simulink model "heat_exchanger_OL"  (R2017b)
settings: Solver=VariableStepAuto  StartTime=0.0  StopTime=200  RelTol=1e-3
values from neighbouring files (symbols this model uses):
  Area = n*A_heat_plate    (= 9.8716)    [heat_exchanger_config.m]    (also in linearization.m = 20)
  cp_H2O = 4190    [heat_exchanger_config.m]    (also in linearization.m)
  cp_wort = 4062    [heat_exchanger_config.m]    (also in linearization.m = 4000)
  HE_delay = 25    [heat_exchanger_config.m]    (also in linearization.m = 5)
  m_H2O = m_wort    (= 10)    [heat_exchanger_config.m]    (also in linearization.m = 1)
  m_wort = 10    [heat_exchanger_config.m]    (also in linearization.m = 1)
  T_H2O_in = 5    [heat_exchanger_config.m]    (also in linearization.m = 10)
  T_wort_in = 95    [heat_exchanger_config.m]    (also in linearization.m = 70)
  U = (m_dot_h_data*cp_wort*(T_wort_in-T_wort_out)*log(Delta_T2/Delta_T1))/     (Area*(Delta_T2-Delta_T1))    [heat_exchanger_config.m]    (also in linearization.m = 1000)
libraries: simulink x1
settings Model: PauseTimes=0  Creator=Alexander  LastModifiedBy=Alexander

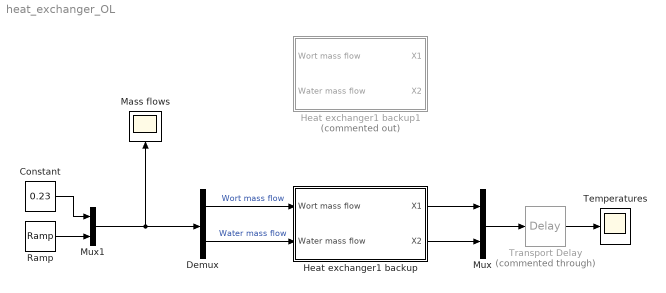
== system heat_exchanger_OL ==
  Constant : Constant  Value=0.23
  Demux : Demux  Outputs=2
  Heat exchanger1 backup : Subsystem
  Heat exchanger1 backup1 : Subsystem  Commented=on
  Mass flows : Scope
  Mux : Mux  Inputs=2
  Mux1 : Mux  Inputs=2
  Ramp : simulink/Sources/Ramp  slope=0.1  start=0  X0=0
  Temperatures : Scope
  Transport Delay : TransportDelay  Commented=through  DelayTime=HE_delay
  wires:
  Transport Delay/1 -> Temperatures/1
  Mux/1 -> Transport Delay/1
  Demux/1 -> Heat exchanger1 backup/1(Wort mass flow)  "Wort mass flow"
  Demux/2 -> Heat exchanger1 backup/2(Water mass flow)  "Water mass flow"
  Constant/1 -> Mux1/1
  Mux1/1 -> Mass flows/1, Demux/1
  Heat exchanger1 backup/1(X1) -> Mux/1
  Heat exchanger1 backup/2(X2) -> Mux/2
  Ramp/1 -> Mux1/2

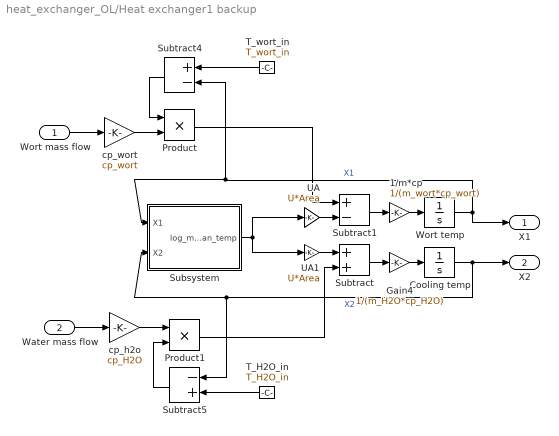
== system heat_exchanger_OL/Heat exchanger1 backup ==
  Wort mass flow : Inport
  Water mass flow : Inport  Port=2
  "1/m*cp " : Gain  Gain=1/(m_wort*cp_wort)
  Cooling temp : Integrator  InitialCondition=T_H2O_in-0.1
  Gain4 : Gain  Gain=1/(m_H2O*cp_H2O)
  Product : Product
  Product1 : Product
  Subsystem : Subsystem
  Subtract : Sum
  Subtract1 : Sum  Inputs=+-
  Subtract4 : Sum  Inputs=+-
  Subtract5 : Sum  Inputs=-+
  T_H2O_in : Constant  Value=T_H2O_in
  T_wort_in : Constant  Value=T_wort_in
  UA : Gain  Gain=U*Area
  "UA1 " : Gain  Gain=U*Area
  Wort temp : Integrator  InitialCondition=T_wort_in-0.1
  cp_h2o : Gain  Gain=cp_H2O
  cp_wort : Gain  Gain=cp_wort
  X1 : Outport
  X2 : Outport  Port=2
  wires:
  Cooling temp/1 -> X2/1, Subtract5/1, Subsystem/2(X2)  "X2"
  "1/m*cp "/1 -> Wort temp/1
  Wort temp/1 -> X1/1, Subsystem/1("X1 "), Subtract4/2  "X1"
  UA/1 -> Subtract1/2
  Subtract1/1 -> "1/m*cp "/1
  Gain4/1 -> Cooling temp/1
  "UA1 "/1 -> Subtract/1
  Subtract/1 -> Gain4/1
  T_wort_in/1 -> Subtract4/1
  Subtract5/1 -> Product1/2
  Product/1 -> Subtract1/1
  T_H2O_in/1 -> Subtract5/2
  Subtract4/1 -> Product/1
  Water mass flow/1 -> cp_h2o/1
  Wort mass flow/1 -> cp_wort/1
  Product1/1 -> Subtract/2
  cp_h2o/1 -> Product1/1
  cp_wort/1 -> Product/2
  Subsystem/1(log_mean_temp) -> UA/1, "UA1 "/1

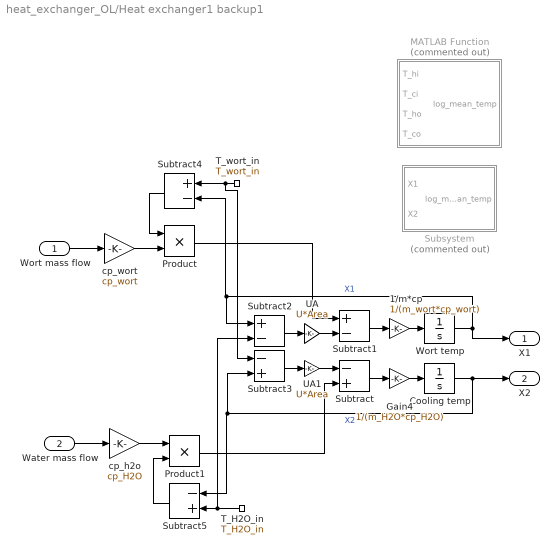
== system heat_exchanger_OL/Heat exchanger1 backup1 ==
  Wort mass flow : Inport
  Water mass flow : Inport  Port=2
  "1/m*cp " : Gain  Gain=1/(m_wort*cp_wort)
  Cooling temp : Integrator  InitialCondition=T_H2O_in-0.1
  Gain4 : Gain  Gain=1/(m_H2O*cp_H2O)
  MATLAB Function : MATLAB Function  Commented=on  TreatAsAtomicUnit=on
  Product : Product
  Product1 : Product
  Subsystem : Subsystem  Commented=on
  Subtract : Sum  Inputs=-+
  Subtract1 : Sum  Inputs=+-
  Subtract2 : Sum  Inputs=+-
  Subtract3 : Sum  Inputs=-+
  Subtract4 : Sum  Inputs=+-
  Subtract5 : Sum  Inputs=-+
  T_H2O_in : Constant  Value=T_H2O_in
  T_wort_in : Constant  Value=T_wort_in
  UA : Gain  Gain=U*Area
  "UA1 " : Gain  Gain=U*Area
  Wort temp : Integrator  InitialCondition=T_wort_in-0.1
  cp_h2o : Gain  Gain=cp_H2O
  cp_wort : Gain  Gain=cp_wort
  X1 : Outport
  X2 : Outport  Port=2
  wires:
  Cooling temp/1 -> X2/1, Subtract3/2, Subtract5/1  "X2"
  "1/m*cp "/1 -> Wort temp/1
  Wort temp/1 -> X1/1, Subtract2/1, Subtract4/2  "X1"
  UA/1 -> Subtract1/2
  Subtract1/1 -> "1/m*cp "/1
  Gain4/1 -> Cooling temp/1
  "UA1 "/1 -> Subtract/1
  Subtract2/1 -> UA/1
  Subtract3/1 -> "UA1 "/1
  Subtract/1 -> Gain4/1
  T_wort_in/1 -> Subtract3/1, Subtract4/1
  Subtract5/1 -> Product1/2
  Product/1 -> Subtract1/1
  T_H2O_in/1 -> Subtract2/2, Subtract5/2
  Subtract4/1 -> Product/1
  Water mass flow/1 -> cp_h2o/1
  Wort mass flow/1 -> cp_wort/1
  Product1/1 -> Subtract/2
  cp_h2o/1 -> Product1/1
  cp_wort/1 -> Product/2

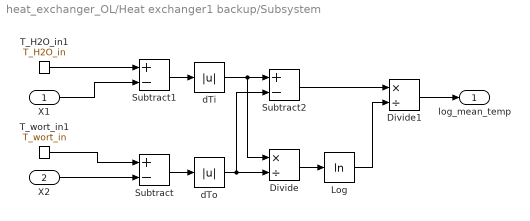
== system heat_exchanger_OL/Heat exchanger1 backup/Subsystem ==
  "X1 " : Inport
  X2 : Inport  Port=2
  Divide : Product  Inputs=*/
  Divide1 : Product  Inputs=*/
  Log : Math  Operator=log  SaturateOnIntegerOverflow=on
  Subtract : Sum  Inputs=+-
  Subtract1 : Sum  Inputs=+-
  Subtract2 : Sum  Inputs=+-
  T_H2O_in1 : Constant  Value=T_H2O_in
  T_wort_in1 : Constant  Value=T_wort_in
  dTi : Abs
  dTo : Abs
  log_mean_temp : Outport
  wires:
  Subtract/1 -> dTo/1
  T_wort_in1/1 -> Subtract/1
  X2/1 -> Subtract/2
  Subtract1/1 -> dTi/1
  "X1 "/1 -> Subtract1/2
  T_H2O_in1/1 -> Subtract1/1
  dTo/1 -> Subtract2/2, Divide/2
  dTi/1 -> Subtract2/1, Divide/1
  Divide/1 -> Log/1
  Log/1 -> Divide1/2
  Divide1/1 -> log_mean_temp/1
  Subtract2/1 -> Divide1/1

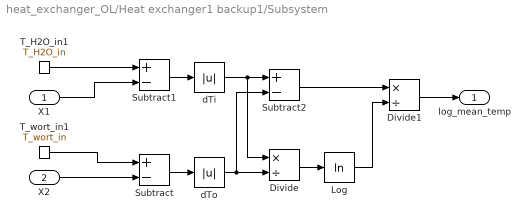
== system heat_exchanger_OL/Heat exchanger1 backup1/Subsystem ==
  "X1 " : Inport
  X2 : Inport  Port=2
  Divide : Product  Inputs=*/
  Divide1 : Product  Inputs=*/
  Log : Math  Operator=log  SaturateOnIntegerOverflow=on
  Subtract : Sum  Inputs=+-
  Subtract1 : Sum  Inputs=+-
  Subtract2 : Sum  Inputs=+-
  T_H2O_in1 : Constant  Value=T_H2O_in
  T_wort_in1 : Constant  Value=T_wort_in
  dTi : Abs
  dTo : Abs
  log_mean_temp : Outport
  wires:
  Subtract/1 -> dTo/1
  T_wort_in1/1 -> Subtract/1
  X2/1 -> Subtract/2
  Subtract1/1 -> dTi/1
  "X1 "/1 -> Subtract1/2
  T_H2O_in1/1 -> Subtract1/1
  dTo/1 -> Subtract2/2, Divide/2
  dTi/1 -> Subtract2/1, Divide/1
  Divide/1 -> Log/1
  Log/1 -> Divide1/2
  Divide1/1 -> log_mean_temp/1
  Subtract2/1 -> Divide1/1

== matlab function heat_exchanger_OL/Heat exchanger1 backup1/MATLAB Function ==
  data: T_hi input; log_mean_temp output; T_ci input; T_ho input; T_co input
function log_mean_temp = fcn(T_hi,T_ci,T_ho,T_co)

dTi=abs(T_hi-T_ci);
dTo=abs(T_ho-T_co);

log_mean_temp = (dTi-dTo)/log(dTi/dTo);

end
